simulink model "decentralized_sat"  (R2023b)
settings: Solver=ode45  StartTime=0.0  StopTime=Tf  RelTol=1e-3
undefined symbols (not defined in the file): Ac_mrs2, Ac_mrs3, b, Bc_mrs2, Bc_mrs3, C2, C3, Cc_mrs2, Cc_mrs3, Dc_mrs2, Dc_mrs3, p01, p02, p03, p04, phi02, phi03, r_pd1, r_pd2, r_pd3, r_pd4, th02, th03, u_max_n1, u_max_n2, u_max_n3, u_max_n4, xc02, xc03
settings Model: Creator=lorenzo  LastModifiedBy=lorenzo

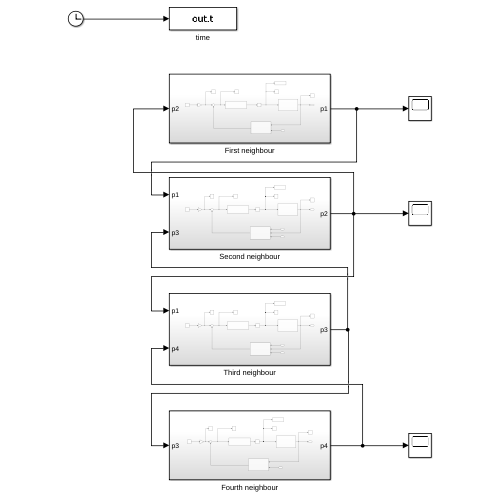
[thumbnail: Simulink's stored preview of the top-level diagram]
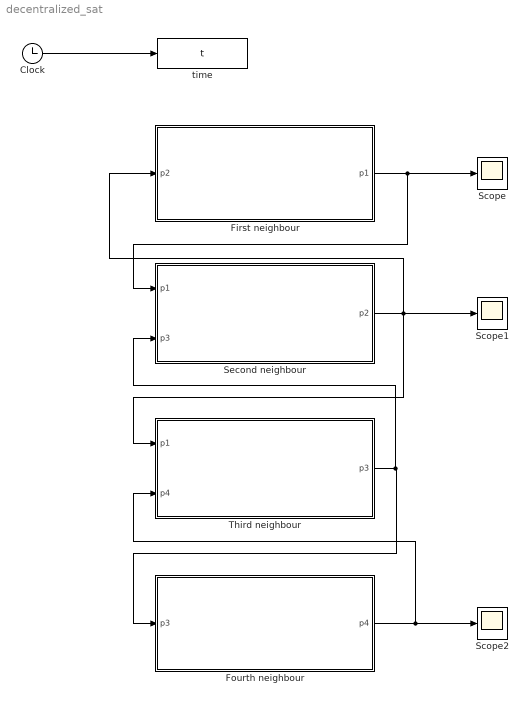
== system decentralized_sat ==
  Clock : Clock
  First neighbour : Subsystem
  Fourth neighbour : Subsystem
  Scope : Scope
  Scope1 : Scope
  Scope2 : Scope
  Second neighbour : Subsystem
  Third neighbour : Subsystem
  time : ToWorkspace  VariableName=t  SampleTime=-1
  wires:
  First neighbour/1(p1) -> Second neighbour/1(p1), Scope/1
  Clock/1 -> time/1
  Second neighbour/1(p2) -> Third neighbour/1(p1), Scope1/1, First neighbour/1(p2)
  Fourth neighbour/1(p4) -> Third neighbour/2(p4), Scope2/1
  Third neighbour/1(p3) -> Second neighbour/2(p3), Fourth neighbour/1(p3)

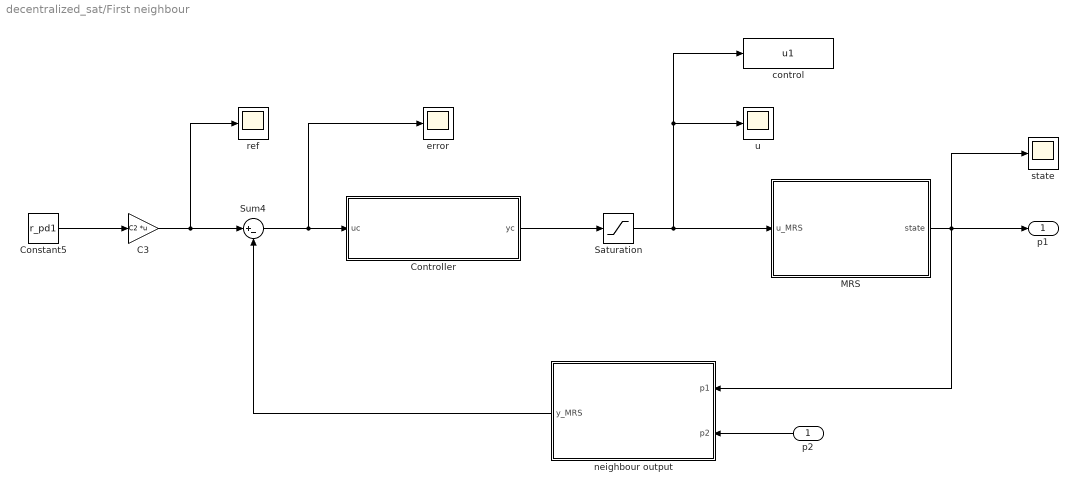
== system decentralized_sat/First neighbour ==
  p2 : Inport
  C3 : Gain  Gain=C2  Multiplication=Matrix(K*u) (u vector)
  Constant5 : Constant  Value=r_pd1  VectorParams1D=off
  Controller : Subsystem
  MRS : Subsystem
  Saturation : Saturate  UpperLimit=u_max_n1  LowerLimit=-u_max_n1
  Sum4 : Sum  Inputs=|+-
  control : ToWorkspace  VariableName=u1  SampleTime=-1
  error : Scope
  neighbour output : Subsystem
  ref : Scope
  state : Scope
  u : Scope
  p1 : Outport
  wires:
  Sum4/1 -> error/1, Controller/1(uc)
  MRS/1(state) -> p1/1, neighbour output/1(p1), state/1
  neighbour output/1(y_MRS) -> Sum4/2
  p2/1 -> neighbour output/2(p2)
  Controller/1(yc) -> Saturation/1
  Saturation/1 -> control/1, u/1, MRS/1(u_MRS)
  Constant5/1 -> C3/1
  C3/1 -> ref/1, Sum4/1

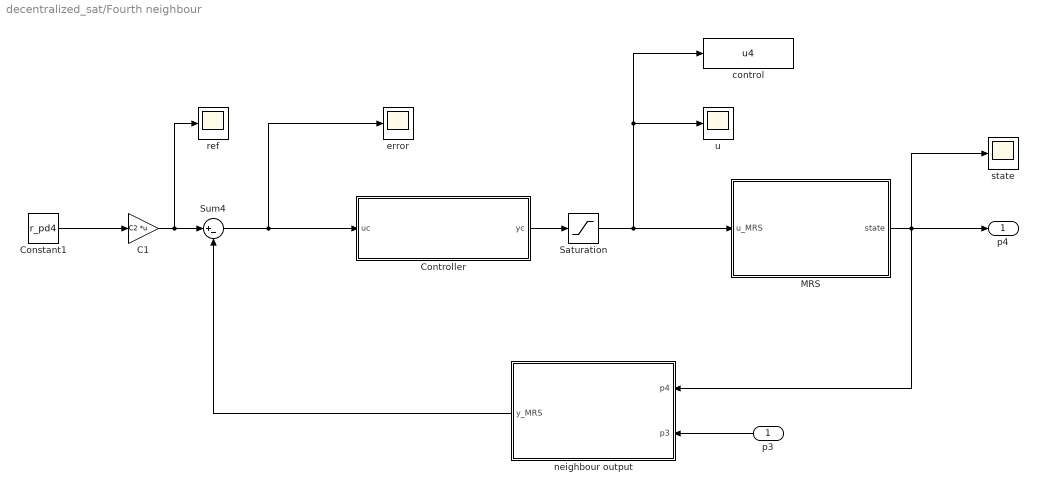
== system decentralized_sat/Fourth neighbour ==
  p3 : Inport
  C1 : Gain  Gain=C2  Multiplication=Matrix(K*u) (u vector)
  Constant1 : Constant  Value=r_pd4  VectorParams1D=off
  Controller : Subsystem
  MRS : Subsystem
  Saturation : Saturate  UpperLimit=u_max_n4  LowerLimit=-u_max_n4
  Sum4 : Sum  Inputs=|+-
  control : ToWorkspace  VariableName=u4  SampleTime=-1
  error : Scope
  neighbour output : Subsystem
  ref : Scope
  state : Scope
  u : Scope
  p4 : Outport
  wires:
  Sum4/1 -> error/1, Controller/1(uc)
  MRS/1(state) -> neighbour output/1(p4), state/1, p4/1
  Controller/1(yc) -> Saturation/1
  neighbour output/1(y_MRS) -> Sum4/2
  p3/1 -> neighbour output/2(p3)
  Constant1/1 -> C1/1
  C1/1 -> ref/1, Sum4/1
  Saturation/1 -> control/1, u/1, MRS/1(u_MRS)

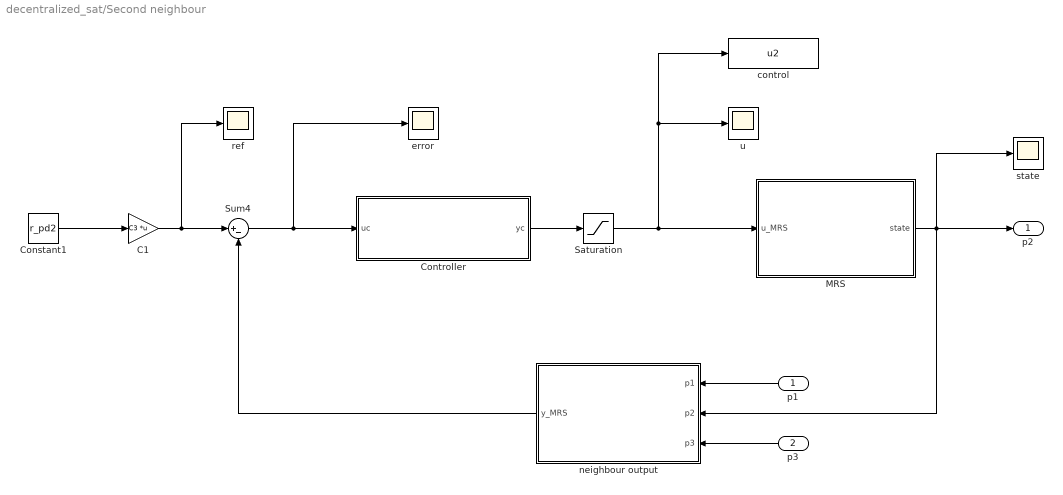
== system decentralized_sat/Second neighbour ==
  p1 : Inport
  p3 : Inport  Port=2
  C1 : Gain  Gain=C3  Multiplication=Matrix(K*u) (u vector)
  Constant1 : Constant  Value=r_pd2  VectorParams1D=off
  Controller : Subsystem
  MRS : Subsystem
  Saturation : Saturate  UpperLimit=u_max_n2  LowerLimit=-u_max_n2
  Sum4 : Sum  Inputs=|+-
  control : ToWorkspace  VariableName=u2  SampleTime=-1
  error : Scope
  neighbour output : Subsystem
  ref : Scope
  state : Scope
  u : Scope
  p2 : Outport
  wires:
  Sum4/1 -> error/1, Controller/1(uc)
  MRS/1(state) -> neighbour output/2(p2), state/1, p2/1
  Controller/1(yc) -> Saturation/1
  neighbour output/1(y_MRS) -> Sum4/2
  p3/1 -> neighbour output/3(p3)
  p1/1 -> neighbour output/1(p1)
  C1/1 -> ref/1, Sum4/1
  Constant1/1 -> C1/1
  Saturation/1 -> control/1, u/1, MRS/1(u_MRS)

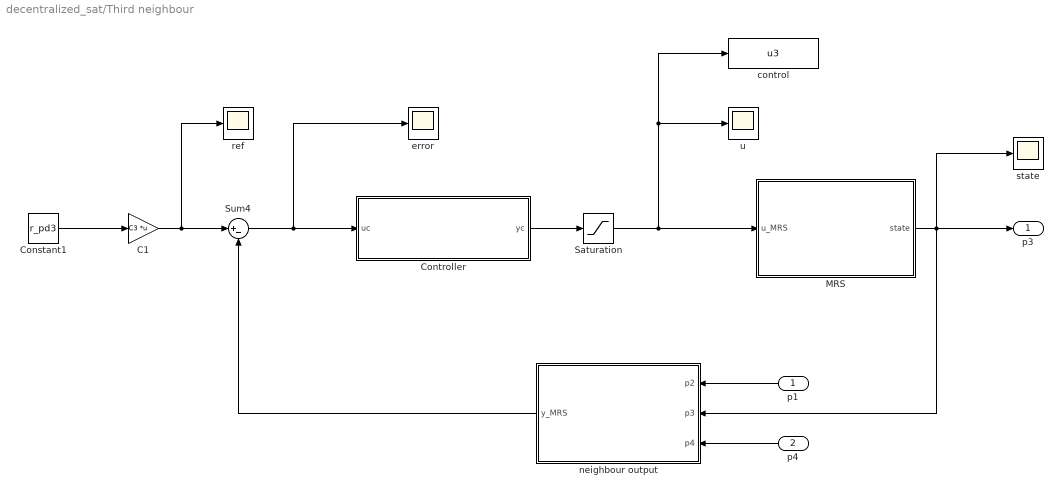
== system decentralized_sat/Third neighbour ==
  p1 : Inport
  p4 : Inport  Port=2
  C1 : Gain  Gain=C3  Multiplication=Matrix(K*u) (u vector)
  Constant1 : Constant  Value=r_pd3  VectorParams1D=off
  Controller : Subsystem
  MRS : Subsystem
  Saturation : Saturate  UpperLimit=u_max_n3  LowerLimit=-u_max_n3
  Sum4 : Sum  Inputs=|+-
  control : ToWorkspace  VariableName=u3  SampleTime=-1
  error : Scope
  neighbour output : Subsystem
  ref : Scope
  state : Scope
  u : Scope
  p3 : Outport
  wires:
  Sum4/1 -> error/1, Controller/1(uc)
  MRS/1(state) -> neighbour output/2(p3), state/1, p3/1
  Controller/1(yc) -> Saturation/1
  neighbour output/1(y_MRS) -> Sum4/2
  p4/1 -> neighbour output/3(p4)
  p1/1 -> neighbour output/1(p2)
  C1/1 -> ref/1, Sum4/1
  Constant1/1 -> C1/1
  Saturation/1 -> control/1, u/1, MRS/1(u_MRS)

== system decentralized_sat/First neighbour/Controller ==
  uc : Inport
  Controller formation : Subsystem
  yc : Outport
  wires:
  uc/1 -> Controller formation/1(uc)
  Controller formation/1(u) -> yc/1

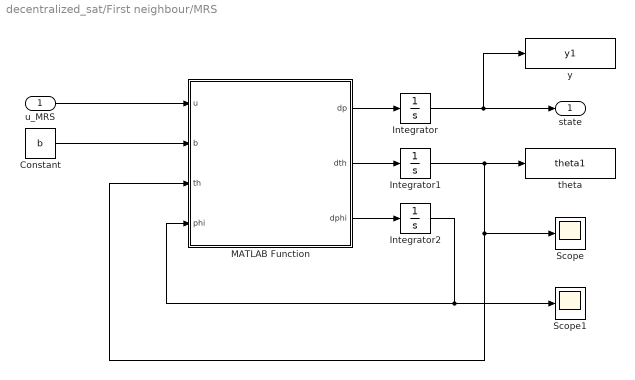
== system decentralized_sat/First neighbour/MRS ==
  u_MRS : Inport
  Constant : Constant  Value=b
  Integrator : Integrator  InitialCondition=p01
  Integrator1 : Integrator  InitialCondition=th02
  Integrator2 : Integrator  InitialCondition=phi02
  MATLAB Function : MATLAB Function  TreatAsAtomicUnit=on
  Scope : Scope
  Scope1 : Scope
  theta : ToWorkspace  VariableName=theta1  SampleTime=-1
  y : ToWorkspace  VariableName=y1  SampleTime=-1
  state : Outport
  wires:
  u_MRS/1 -> MATLAB Function/1(u)
  Constant/1 -> MATLAB Function/2(b)
  MATLAB Function/2(dth) -> Integrator1/1
  MATLAB Function/1(dp) -> Integrator/1
  Integrator1/1 -> MATLAB Function/3(th), Scope/1, theta/1
  MATLAB Function/3(dphi) -> Integrator2/1
  Integrator2/1 -> Scope1/1, MATLAB Function/4(phi)
  Integrator/1 -> y/1, state/1

== system decentralized_sat/First neighbour/neighbour output ==
  p1 : Inport
  p2 : Inport  Port=2
  C : Gain  Gain=C2  Multiplication=Matrix(K*u) (u vector)
  MATLAB Function : MATLAB Function  TreatAsAtomicUnit=on
  y_MRS : Outport
  wires:
  C/1 -> y_MRS/1
  p1/1 -> MATLAB Function/1(y1)
  p2/1 -> MATLAB Function/2(y2)
  MATLAB Function/1(yn) -> C/1

== system decentralized_sat/Fourth neighbour/Controller ==
  uc : Inport
  Controller formation : Subsystem
  yc : Outport
  wires:
  uc/1 -> Controller formation/1(uc)
  Controller formation/1(u) -> yc/1

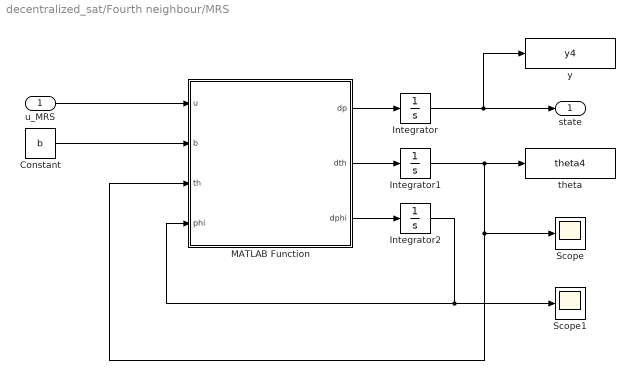
== system decentralized_sat/Fourth neighbour/MRS ==
  u_MRS : Inport
  Constant : Constant  Value=b
  Integrator : Integrator  InitialCondition=p04
  Integrator1 : Integrator  InitialCondition=th03
  Integrator2 : Integrator  InitialCondition=phi03
  MATLAB Function : MATLAB Function  TreatAsAtomicUnit=on
  Scope : Scope
  Scope1 : Scope
  theta : ToWorkspace  VariableName=theta4  SampleTime=-1
  y : ToWorkspace  VariableName=y4  SampleTime=-1
  state : Outport
  wires:
  u_MRS/1 -> MATLAB Function/1(u)
  Constant/1 -> MATLAB Function/2(b)
  MATLAB Function/2(dth) -> Integrator1/1
  MATLAB Function/1(dp) -> Integrator/1
  Integrator1/1 -> MATLAB Function/3(th), Scope/1, theta/1
  MATLAB Function/3(dphi) -> Integrator2/1
  Integrator2/1 -> Scope1/1, MATLAB Function/4(phi)
  Integrator/1 -> y/1, state/1

== system decentralized_sat/Fourth neighbour/neighbour output ==
  p4 : Inport
  p3 : Inport  Port=2
  C : Gain  Gain=C2  Multiplication=Matrix(K*u) (u vector)
  MATLAB Function : MATLAB Function  TreatAsAtomicUnit=on
  y_MRS : Outport
  wires:
  C/1 -> y_MRS/1
  MATLAB Function/1(yn) -> C/1
  p3/1 -> MATLAB Function/1(y1)
  p4/1 -> MATLAB Function/2(y2)

== system decentralized_sat/Second neighbour/Controller ==
  uc : Inport
  Controller formation : Subsystem
  yc : Outport
  wires:
  uc/1 -> Controller formation/1(uc)
  Controller formation/1(u) -> yc/1

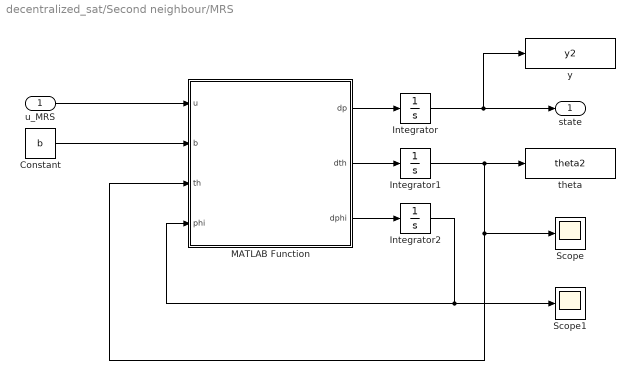
== system decentralized_sat/Second neighbour/MRS ==
  u_MRS : Inport
  Constant : Constant  Value=b
  Integrator : Integrator  InitialCondition=p02
  Integrator1 : Integrator  InitialCondition=th02
  Integrator2 : Integrator  InitialCondition=phi02
  MATLAB Function : MATLAB Function  TreatAsAtomicUnit=on
  Scope : Scope
  Scope1 : Scope
  theta : ToWorkspace  VariableName=theta2  SampleTime=-1
  y : ToWorkspace  VariableName=y2  SampleTime=-1
  state : Outport
  wires:
  u_MRS/1 -> MATLAB Function/1(u)
  Constant/1 -> MATLAB Function/2(b)
  MATLAB Function/2(dth) -> Integrator1/1
  MATLAB Function/1(dp) -> Integrator/1
  Integrator1/1 -> MATLAB Function/3(th), Scope/1, theta/1
  MATLAB Function/3(dphi) -> Integrator2/1
  Integrator2/1 -> Scope1/1, MATLAB Function/4(phi)
  Integrator/1 -> y/1, state/1

== system decentralized_sat/Second neighbour/neighbour output ==
  p1 : Inport
  p2 : Inport  Port=2
  p3 : Inport  Port=3
  C : Gain  Gain=C3  Multiplication=Matrix(K*u) (u vector)
  MATLAB Function : MATLAB Function  TreatAsAtomicUnit=on
  y_MRS : Outport
  wires:
  C/1 -> y_MRS/1
  MATLAB Function/1(yn) -> C/1
  p3/1 -> MATLAB Function/3(y3)
  p2/1 -> MATLAB Function/2(y2)
  p1/1 -> MATLAB Function/1(y1)

== system decentralized_sat/Third neighbour/Controller ==
  uc : Inport
  Controller formation : Subsystem
  yc : Outport
  wires:
  uc/1 -> Controller formation/1(uc)
  Controller formation/1(u) -> yc/1

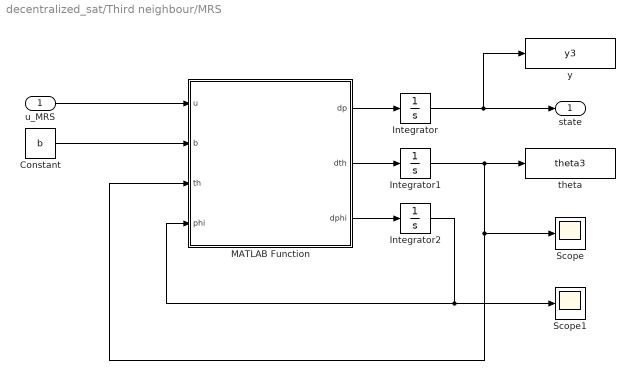
== system decentralized_sat/Third neighbour/MRS ==
  u_MRS : Inport
  Constant : Constant  Value=b
  Integrator : Integrator  InitialCondition=p03
  Integrator1 : Integrator  InitialCondition=th03
  Integrator2 : Integrator  InitialCondition=phi03
  MATLAB Function : MATLAB Function  TreatAsAtomicUnit=on
  Scope : Scope
  Scope1 : Scope
  theta : ToWorkspace  VariableName=theta3  SampleTime=-1
  y : ToWorkspace  VariableName=y3  SampleTime=-1
  state : Outport
  wires:
  u_MRS/1 -> MATLAB Function/1(u)
  Constant/1 -> MATLAB Function/2(b)
  MATLAB Function/2(dth) -> Integrator1/1
  MATLAB Function/1(dp) -> Integrator/1
  Integrator1/1 -> MATLAB Function/3(th), Scope/1, theta/1
  MATLAB Function/3(dphi) -> Integrator2/1
  Integrator2/1 -> Scope1/1, MATLAB Function/4(phi)
  Integrator/1 -> y/1, state/1

== system decentralized_sat/Third neighbour/neighbour output ==
  p2 : Inport
  p3 : Inport  Port=2
  p4 : Inport  Port=3
  C : Gain  Gain=C3  Multiplication=Matrix(K*u) (u vector)
  MATLAB Function : MATLAB Function  TreatAsAtomicUnit=on
  y_MRS : Outport
  wires:
  C/1 -> y_MRS/1
  MATLAB Function/1(yn) -> C/1
  p4/1 -> MATLAB Function/3(y3)
  p3/1 -> MATLAB Function/2(y2)
  p2/1 -> MATLAB Function/1(y1)

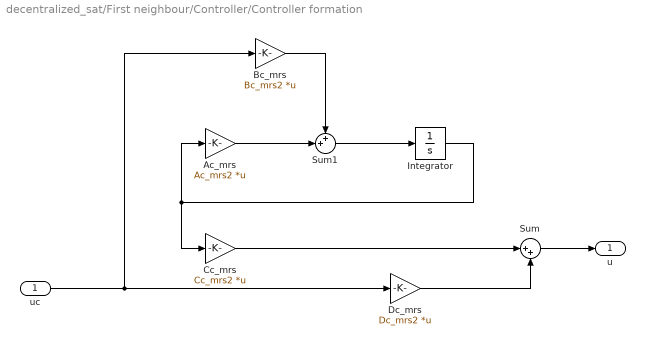
== system decentralized_sat/First neighbour/Controller/Controller formation ==
  uc : Inport
  Ac_mrs : Gain  Gain=Ac_mrs2  Multiplication=Matrix(K*u) (u vector)
  Bc_mrs : Gain  Gain=Bc_mrs2  Multiplication=Matrix(K*u) (u vector)
  Cc_mrs : Gain  Gain=Cc_mrs2  Multiplication=Matrix(K*u) (u vector)
  Dc_mrs : Gain  Gain=Dc_mrs2  Multiplication=Matrix(K*u) (u vector)
  Integrator : Integrator  InitialCondition=xc02
  Sum : Sum  Inputs=|++
  Sum1 : Sum  Inputs=++|
  u : Outport
  wires:
  Bc_mrs/1 -> Sum1/1
  Cc_mrs/1 -> Sum/1
  uc/1 -> Bc_mrs/1, Dc_mrs/1
  Integrator/1 -> Ac_mrs/1, Cc_mrs/1
  Dc_mrs/1 -> Sum/2
  Sum/1 -> u/1
  Ac_mrs/1 -> Sum1/2
  Sum1/1 -> Integrator/1

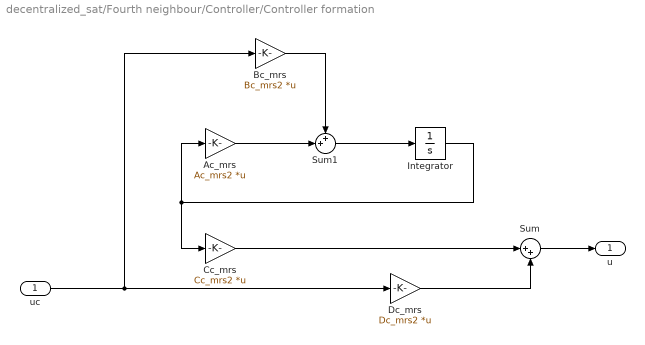
== system decentralized_sat/Fourth neighbour/Controller/Controller formation ==
  uc : Inport
  Ac_mrs : Gain  Gain=Ac_mrs2  Multiplication=Matrix(K*u) (u vector)
  Bc_mrs : Gain  Gain=Bc_mrs2  Multiplication=Matrix(K*u) (u vector)
  Cc_mrs : Gain  Gain=Cc_mrs2  Multiplication=Matrix(K*u) (u vector)
  Dc_mrs : Gain  Gain=Dc_mrs2  Multiplication=Matrix(K*u) (u vector)
  Integrator : Integrator  InitialCondition=xc02
  Sum : Sum  Inputs=|++
  Sum1 : Sum  Inputs=++|
  u : Outport
  wires:
  Bc_mrs/1 -> Sum1/1
  Cc_mrs/1 -> Sum/1
  uc/1 -> Bc_mrs/1, Dc_mrs/1
  Integrator/1 -> Ac_mrs/1, Cc_mrs/1
  Dc_mrs/1 -> Sum/2
  Sum/1 -> u/1
  Ac_mrs/1 -> Sum1/2
  Sum1/1 -> Integrator/1

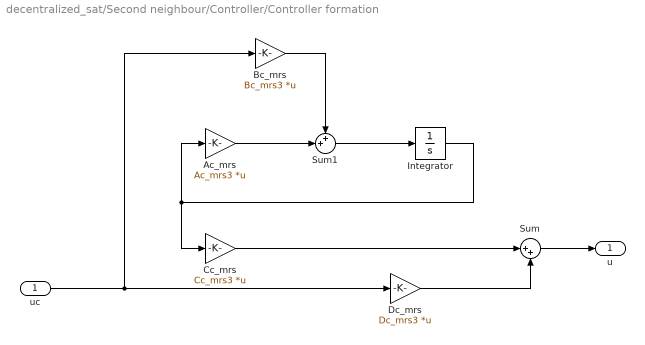
== system decentralized_sat/Second neighbour/Controller/Controller formation ==
  uc : Inport
  Ac_mrs : Gain  Gain=Ac_mrs3  Multiplication=Matrix(K*u) (u vector)
  Bc_mrs : Gain  Gain=Bc_mrs3  Multiplication=Matrix(K*u) (u vector)
  Cc_mrs : Gain  Gain=Cc_mrs3  Multiplication=Matrix(K*u) (u vector)
  Dc_mrs : Gain  Gain=Dc_mrs3  Multiplication=Matrix(K*u) (u vector)
  Integrator : Integrator  InitialCondition=xc03
  Sum : Sum  Inputs=|++
  Sum1 : Sum  Inputs=++|
  u : Outport
  wires:
  Bc_mrs/1 -> Sum1/1
  Cc_mrs/1 -> Sum/1
  uc/1 -> Bc_mrs/1, Dc_mrs/1
  Integrator/1 -> Ac_mrs/1, Cc_mrs/1
  Dc_mrs/1 -> Sum/2
  Sum/1 -> u/1
  Ac_mrs/1 -> Sum1/2
  Sum1/1 -> Integrator/1

== system decentralized_sat/Third neighbour/Controller/Controller formation ==
  uc : Inport
  Ac_mrs : Gain  Gain=Ac_mrs3  Multiplication=Matrix(K*u) (u vector)
  Bc_mrs : Gain  Gain=Bc_mrs3  Multiplication=Matrix(K*u) (u vector)
  Cc_mrs : Gain  Gain=Cc_mrs3  Multiplication=Matrix(K*u) (u vector)
  Dc_mrs : Gain  Gain=Dc_mrs3  Multiplication=Matrix(K*u) (u vector)
  Integrator : Integrator  InitialCondition=xc03
  Sum : Sum  Inputs=|++
  Sum1 : Sum  Inputs=++|
  u : Outport
  wires:
  Bc_mrs/1 -> Sum1/1
  Cc_mrs/1 -> Sum/1
  uc/1 -> Bc_mrs/1, Dc_mrs/1
  Integrator/1 -> Ac_mrs/1, Cc_mrs/1
  Dc_mrs/1 -> Sum/2
  Sum/1 -> u/1
  Ac_mrs/1 -> Sum1/2
  Sum1/1 -> Integrator/1

== matlab function decentralized_sat/Third neighbour/MRS/MATLAB Function ==
  data: u input; b input; dp output; th input; dth output; phi input; dphi output
function [dp,dth,dphi] = platoon_MRS(u,b,th,phi)

ui = u(3:4);

th1 = th(1);

phi1 = phi(1);

B = eye(2);

Bth = tan(phi1)*[cos(th1) sin(th1)];

Bphi = 1/b*[-sin(th1) cos(th1)];

dp = B*ui;
dth = Bth*ui;
dphi = Bphi*ui;

== matlab function decentralized_sat/First neighbour/MRS/MATLAB Function ==
  data: u input; b input; dp output; th input; dth output; phi input; dphi output
function [dp,dth,dphi] = platoon_MRS(u,b,th,phi)

ui = u(1:2);

th1 = th(1);

phi1 = phi(1);

B = eye(2);

Bth = tan(phi1)*[cos(th1) sin(th1)];

Bphi = 1/b*[-sin(th1) cos(th1)];

dp = B*ui;
dth = Bth*ui;
dphi = Bphi*ui;

== matlab function decentralized_sat/Third neighbour/neighbour output/MATLAB Function ==
  data: y1 input; yn output; y2 input; y3 input
function yn = fcn(y1,y2,y3)

yn = [y1;y2;y3];

== matlab function decentralized_sat/Second neighbour/MRS/MATLAB Function ==
  data: u input; b input; dp output; th input; dth output; phi input; dphi output
function [dp,dth,dphi] = platoon_MRS(u,b,th,phi)

ui = u(3:4);

th1 = th(1);

phi1 = phi(1);

B = eye(2);

Bth = tan(phi1)*[cos(th1) sin(th1)];

Bphi = 1/b*[-sin(th1) cos(th1)];

dp = B*ui;
dth = Bth*ui;
dphi = Bphi*ui;

== matlab function decentralized_sat/Second neighbour/neighbour output/MATLAB Function ==
  data: y1 input; yn output; y2 input; y3 input
function yn = fcn(y1,y2,y3)

yn = [y1;y2;y3];

== matlab function decentralized_sat/Fourth neighbour/MRS/MATLAB Function ==
  data: u input; b input; dp output; th input; dth output; phi input; dphi output
function [dp,dth,dphi] = platoon_MRS(u,b,th,phi)

ui = u(3:4);

th1 = th(1);

phi1 = phi(1);

B = eye(2);

Bth = tan(phi1)*[cos(th1) sin(th1)];

Bphi = 1/b*[-sin(th1) cos(th1)];

dp = B*ui;
dth = Bth*ui;
dphi = Bphi*ui;

== matlab function decentralized_sat/Fourth neighbour/neighbour output/MATLAB Function ==
  data: y1 input; yn output; y2 input
function yn = fcn(y1,y2)

yn = [y1;y2];

== matlab function decentralized_sat/First neighbour/neighbour output/MATLAB Function ==
  data: y1 input; yn output; y2 input
function yn = fcn(y1,y2)

yn = [y1;y2];
